simulink model "OFDMA_Simulink_Demo"  (R2016a)
settings: Solver=FixedStepDiscrete  StartTime=0.0  StopTime=10  RelTol=1e-3
InitFcn:
  | init_ofdma
values from neighbouring files (symbols this model uses):
  FFTLength = numUsers * Nsc    (= 64)    [init_ofdma.m]
  Nsc = 16    [init_ofdma.m]
  numUsers = 4    [init_ofdma.m]
libraries: commdigbbndpm3 x10, commsink2 x5, dspxfrm3 x2, commchan3 x1
settings Model: Creator=ASUS  LastModifiedBy=ASUS

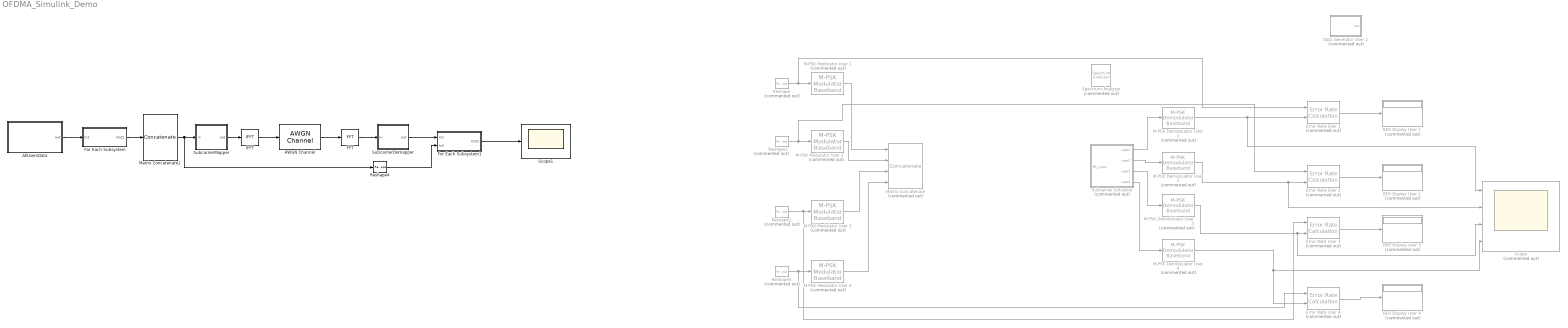
== system OFDMA_Simulink_Demo ==
  AWGN Channel : commchan3/AWGN Channel  InputProcessing=Columns as channels (frame based)  seed=67  noiseMode="Signal to noise ratio  (Eb/No)"  EbNodB=EbNo  EsNodB=10  SNRdB=10  bitsPerSym=2  Ps=1  Tsym=1  variance=1
  AllUsersData : MATLAB Function  TreatAsAtomicUnit=on
  BER Display User {1..4} (4 alike) : Display  Commented=on
  Data Generator User 2 : MATLAB Function  Commented=on  TreatAsAtomicUnit=on
  Error Rate User {1..4} (4 alike) : commsink2/Error Rate Calculation  Commented=on  N=0  st_delay=0  cp_mode=Entire frame  subframe=[]  PMode=Port  WsName=ErrorVec  RsMode2=off  stop=off  numErr=100  maxBits=1e6
  FFT : dspxfrm3/FFT  FFTImplementation=Auto  CompMethod=Table lookup  TableOpt=NEW  TableOptActive=Speed  BitRevOrder=off  Normalize=off  InheritFFTLength=off  FFTLength=FFTLength  WrapInput=on  roundingMode=Floor  overflowMode=off  firstCoeffDataTypeStr=Inherit: Same word length as input  firstCoeffLastDataTypeStr=Inherit: Same word length as input  outputMin=[]  outputMax=[]
  For Each Subsystem : Subsystem  TreatAsAtomicUnit=on
  For Each Subsystem1 : Subsystem  TreatAsAtomicUnit=on
  IFFT : dspxfrm3/IFFT  FFTImplementation=Auto  CompMethod=Table lookup  TableOpt=NEW  TableOptActive=Speed  BitRevOrder=off  cs_in=off  Normalize=on  InheritFFTLength=off  FFTLength=FFTLength  WrapInput=on  mode=Complex  outSamplingMode=Sample based  roundingMode=Floor  overflowMode=off  firstCoeffDataTypeStr=Inherit: Same word length as input  firstCoeffLastDataTypeStr=Inherit: Same word length as input  outputMin=[]  outputMax=[]
  M-PSK Demodulator User {1..4} (4 alike) : commdigbbndpm3/M-PSK Demodulator Baseband  Commented=on  M=4  OutType=Integer  DecType=Hard decision  VarSource=Dialog  Variance=1  Dec=Gray  Mapping=[0:7]  Ph=0  outDtype1=Inherit via internal rule  outDtype2=Inherit via internal rule  derotateFactorWordLen=16  derotateFactorDataTypeStr=Inherit: Same word length as input  derotateFactorLastDataTypeStr=Inherit: Same word length as input
  M-PSK Modulator User {1..4} (4 alike) : commdigbbndpm3/M-PSK Modulator Baseband  Commented=on  M=4  InType=Integer  Enc=Gray  Mapping=[0:7]  Ph=0  outDtype=double  outWordLen=16  outUDDataType=sfix(16)  outFracLenMode=Best precision  outFracLen=15  outDataTypeStr=double  outLastDataTypeStr=double
  Matrix Concatenate : Concatenate  Commented=on  NumInputs=4  Mode=Multidimensional array
  Matrix Concatenate1 : Concatenate  NumInputs=1
  Reshape{,1..3} (4 alike) : Reshape  Commented=on  OutputDimensionality=Customize  OutputDimensions=[20, 1]
  Reshape4 : Reshape  OutputDimensionality=Customize  OutputDimensions=[4 16]
  Scope : Scope  Commented=on  NumInputPorts=4
  Scope1 : Scope
  Spectrum Analyzer : SpectrumAnalyzer  Commented=on
  Subcarrier Extractor : MATLAB Function  Commented=on  TreatAsAtomicUnit=on
  SubcarrierDemapper : MATLAB Function  TreatAsAtomicUnit=on
  SubcarrierMapper : MATLAB Function  TreatAsAtomicUnit=on
  wires:
  M-PSK Modulator User 1/1 -> Matrix Concatenate/1
  M-PSK Demodulator User 1/1 -> Error Rate User 1/2, Scope/1
  Reshape/1 -> Error Rate User 1/1, M-PSK Modulator User 1/1
  AWGN Channel/1 -> FFT/1
  IFFT/1 -> AWGN Channel/1
  Error Rate User 1/1 -> BER Display User 1/1
  Reshape1/1 -> Error Rate User 2/1, M-PSK Modulator User 2/1
  Reshape2/1 -> Error Rate User 3/1, M-PSK Modulator User 3/1
  Reshape3/1 -> Error Rate User 4/1, M-PSK Modulator User 4/1
  M-PSK Modulator User 2/1 -> Matrix Concatenate/2
  M-PSK Modulator User 3/1 -> Matrix Concatenate/3
  M-PSK Modulator User 4/1 -> Matrix Concatenate/4
  Subcarrier Extractor/2(user2) -> M-PSK Demodulator User 2/1
  Subcarrier Extractor/1(user1) -> M-PSK Demodulator User 1/1
  Subcarrier Extractor/3(user3) -> M-PSK Demodulator User 3/1
  Subcarrier Extractor/4(user4) -> M-PSK Demodulator User 4/1
  M-PSK Demodulator User 4/1 -> Error Rate User 4/2, Scope/4
  M-PSK Demodulator User 3/1 -> Scope/3, Error Rate User 3/2
  M-PSK Demodulator User 2/1 -> Scope/2, Error Rate User 2/2
  Error Rate User 2/1 -> BER Display User 2/1
  Error Rate User 3/1 -> BER Display User 3/1
  Error Rate User 4/1 -> BER Display User 4/1
  AllUsersData/1(out) -> For Each Subsystem/1(In1)
  For Each Subsystem/1(Out1) -> Matrix Concatenate1/1
  Matrix Concatenate1/1 -> Reshape4/1, SubcarrierMapper/1(in)
  SubcarrierMapper/1(out) -> IFFT/1
  FFT/1 -> SubcarrierDemapper/1(in)
  SubcarrierDemapper/1(out) -> For Each Subsystem1/1(In1)
  For Each Subsystem1/1(Out1) -> Scope1/1
  Reshape4/1 -> For Each Subsystem1/2(In2)

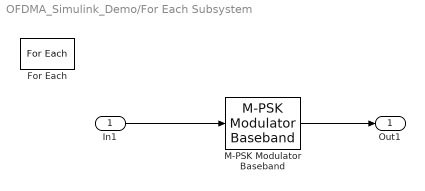
== system OFDMA_Simulink_Demo/For Each Subsystem ==
  In1 : Inport  Partition=on  PartitionDimension=2  PartitionWidth=1
  For Each : ForEach  DisableCoverage=on  IndexMode=One-based
  M-PSK Modulator Baseband : commdigbbndpm3/M-PSK Modulator Baseband  M=4  InType=Integer  Enc=Gray  Mapping=[0:7]  Ph=0  outDtype=double  outWordLen=16  outUDDataType=sfix(16)  outFracLenMode=Best precision  outFracLen=15  outDataTypeStr=double  outLastDataTypeStr=double
  Out1 : Outport  ConcatenationDimension=1
  wires:
  In1/1 -> M-PSK Modulator Baseband/1
  M-PSK Modulator Baseband/1 -> Out1/1

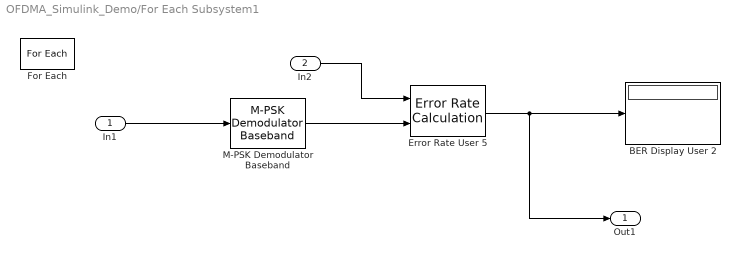
== system OFDMA_Simulink_Demo/For Each Subsystem1 ==
  In1 : Inport  Partition=on  PartitionDimension=2  PartitionWidth=1
  In2 : Inport  Port=2  Partition=on  PartitionDimension=2  PartitionWidth=1
  BER Display User 2 : Display
  Error Rate User 5 : commsink2/Error Rate Calculation  N=0  st_delay=0  cp_mode=Entire frame  subframe=[]  PMode=Port  WsName=ErrorVec  RsMode2=off  stop=off  numErr=100  maxBits=1e6
  For Each : ForEach  DisableCoverage=on  IndexMode=One-based
  M-PSK Demodulator Baseband : commdigbbndpm3/M-PSK Demodulator Baseband  M=4  OutType=Integer  DecType=Hard decision  VarSource=Dialog  Variance=1  Dec=Gray  Mapping=[0:7]  Ph=0  outDtype1=Inherit via internal rule  outDtype2=Inherit via internal rule  derotateFactorWordLen=16  derotateFactorDataTypeStr=Inherit: Same word length as input  derotateFactorLastDataTypeStr=Inherit: Same word length as input
  Out1 : Outport  ConcatenationDimension=1
  wires:
  In1/1 -> M-PSK Demodulator Baseband/1
  M-PSK Demodulator Baseband/1 -> Error Rate User 5/2
  In2/1 -> Error Rate User 5/1
  Error Rate User 5/1 -> Out1/1, BER Display User 2/1

== matlab function OFDMA_Simulink_Demo/Subcarrier Extractor ==
  data: fft_input input; user1 output size=[20, 1]; user2 output size=[20, 1]; user3 output size=[20, 1]; user4 output size=[20, 1]
function [user1, user2, user3, user4] = fcn(fft_input)
% Extract subcarriers for each of 4 users
% Input: fft_input [80x1] - all subcarriers from FFT
% Outputs: 4 users, each [20x1] - their allocated subcarriers

% Convert input to column vector (handles any dimension)
fft_col = fft_input(:);

% Extract each user's allocated subcarriers
user1 = fft_col(1:20);    % User 1: subcarriers 1-20
user2 = fft_col(21:40);   % User 2: subcarriers 21-40
user3 = fft_col(41:60);   % User 3: subcarriers 41-60
user4 = fft_col(61:80);   % User 4: subcarriers 61-80
end

== matlab function OFDMA_Simulink_Demo/AllUsersData ==
  data: out output double size=[numUsers Nsc]; numUsers parameter double size=1; Nsc parameter double size=1
function out = AllUsersData(numUsers, Nsc)

% FORCE FIXED SIZE OUTPUT
out = complex(zeros(4,16));   % <-- hardcode once to stabilize model

% generate random QPSK data per user
for u = 1:16
    bits = randi([0 3],4,1);
    out(:,u) = pskmod(bits,4,pi/4);
end

== matlab function OFDMA_Simulink_Demo/Data Generator User 2 ==
  data: out output double size=[20 1]
function out = fcn()

N_SC = 20;
out = double(randi([0 3], N_SC, 1));

end

%numUsers * subcarriersPerUser

== matlab function OFDMA_Simulink_Demo/SubcarrierMapper ==
  data: in input; out output double size=[FFTLength 1]; numUsers parameter size=1; Nsc parameter size=1; FFTLength parameter size=1
function out = SubcarrierMapper(in, numUsers, Nsc, FFTLength)

% ---- FORCE FIXED SIZE OUTPUT ----
out = complex(zeros(64,1));
% in = [numUsers × Nsc] symbols
% Map each user to its OFDMA subcarriers

idx = 1;

for u = 1:numUsers
    for k = 1:Nsc
        out(idx) = in(u,k);
        idx = idx + 1;
    end
end

== matlab function OFDMA_Simulink_Demo/SubcarrierDemapper ==
  data: in input; out output double size=[numUsers Nsc]; numUsers parameter size=1; Nsc parameter size=1
function out = SubcarrierDemapper(in, numUsers, Nsc)

out = complex(zeros(4,16));

idx = 1;

for u = 1:numUsers
    for k = 1:Nsc
        out(u,k) = in(idx);
        idx = idx + 1;
    end
end
